simulink model "problem_1_sim"  (R2025a)
settings: Solver=VariableStepAuto  StartTime=0.0  StopTime=t_sim  RelTol=1e-3
values from neighbouring files (symbols this model uses):
  C = [1 0]    [problem_1.m]
  md = MPCInit(Ad,Bd,Cy,Cz,Dz,Cc,Dc,Hp,Hw,zblk,Hc,ublk,   		      du_max,du_min,u_max,u_min,z_max,   		      z_min,Q,R,[],[],Ts,0,'qp_as')    [problem_1.m]
  r = 1    [problem_1.m]
  Ts = 0.05    [problem_1.m]
libraries: cstblocks x1
settings Model: Creator=s360159  LastModifiedBy=s360159

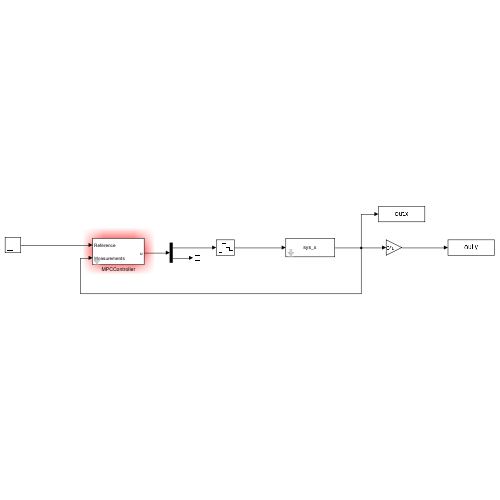
[thumbnail: Simulink's stored preview of the top-level diagram]
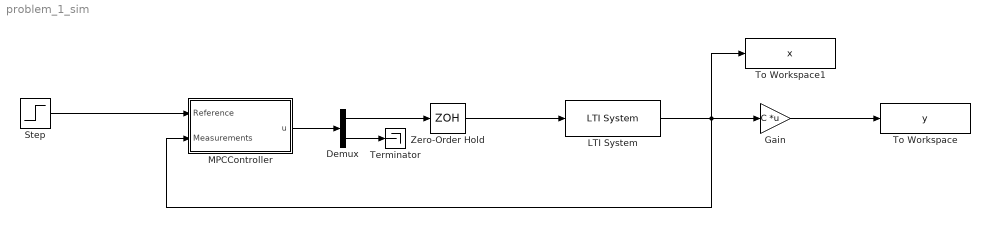
== system problem_1_sim ==
  Demux : Demux  Outputs=2
  Gain : Gain  Gain=C  Multiplication=Matrix(K*u)
  LTI System : cstblocks/LTI System  sys=sys_x  IC=[]  PadeOrder=0
  MPCController : Subsystem  mask{md=md}
      mask prompts: md "MPCData"
  Step : Step  Time=0  After=r  SampleTime=Ts
  Terminator : Terminator
  To Workspace : ToWorkspace  VariableName=y  SaveFormat=Timeseries  SampleTime=Ts
  To Workspace1 : ToWorkspace  VariableName=x  SaveFormat=Timeseries  SampleTime=Ts
  Zero-Order Hold : ZeroOrderHold  SampleTime=Ts
  wires:
  Step/1 -> MPCController/1(Reference)
  MPCController/1(u) -> Demux/1
  Demux/2 -> Terminator/1
  Demux/1 -> Zero-Order Hold/1
  Zero-Order Hold/1 -> LTI System/1
  LTI System/1 -> To Workspace1/1, MPCController/2(Measurements), Gain/1
  Gain/1 -> To Workspace/1

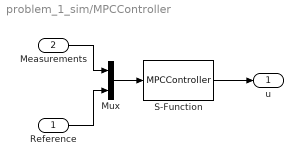
== system problem_1_sim/MPCController ==
  Reference : Inport
  Measurements : Inport  Port=2
  Mux : Mux  Inputs=2
  S-Function : S-Function  FunctionName=MPCController  Parameters=md  SFunctionDeploymentMode=off  EnableBusSupport=off
  u : Outport
  wires:
  Mux/1 -> S-Function/1
  Measurements/1 -> Mux/1
  Reference/1 -> Mux/2
  S-Function/1 -> u/1
